simulink model "Step_03"  (Simulink 7.9)
settings: Solver=ode23  StartTime=0.0  StopTime=100  MaxStep=1  RelTol=1e-3
libraries: simulink x1
settings Model: Creator=wcampbel  LastModifiedBy=wcampbel
settings DebuggingCC: FcnCallInpInsideContextMsg=Use local settings  StrictBusMsg=Warning
settings GRTTargetCC: CombineOutputUpdateFcns=off  GRTInterface=on

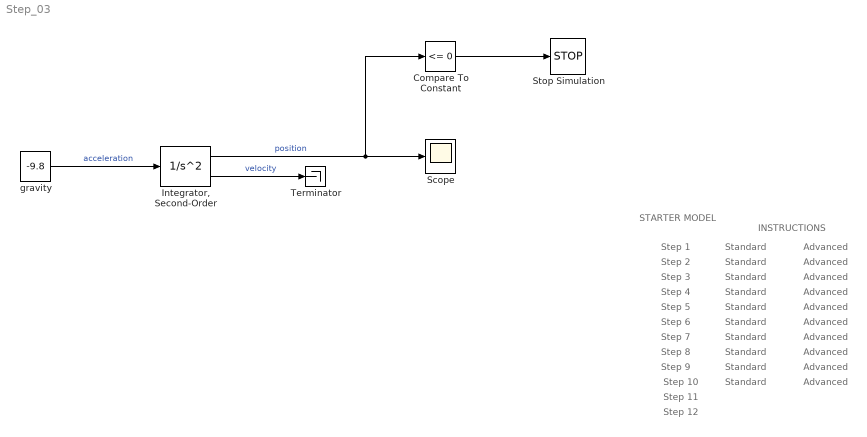
== system Step_03 ==
  note: Step 1
  note: Step 2
  note: Step 3
  note: STARTER
      | MODEL
  note: INSTRUCTIONS
  note: Step 4
  note: Step 5
  note: Step 6
  note: Standard
  note: Advanced
  note: Standard
  note: Advanced
  note: Standard
  note: Advanced
  note: Standard
  note: Standard
  note: Advanced
  note: Standard
  note: Advanced
  note: Step 7
  note: Step 8
  note: Step 9
  note: Step 10
  note: Step 11
  note: Standard
  note: Advanced
  note: Advanced
  note: Advanced
  note: Advanced
  note: Standard
  note: Standard
  note: Standard
  note: Advanced
  note: Step 12
  Compare To Constant : simulink/Logic and Bit Operations/Compare To Constant  relop=<=  const=0  OutDataTypeStr=boolean
  "Integrator, Second-Order" : SecondOrderIntegrator  ICX=500  ICDXDT=5
  Scope : Scope
      settings: TimeRange=12  YMin=-100  YMax=600
  Stop Simulation : Stop
  Terminator : Terminator
  gravity : Constant  Value=-9.8
  wires:
  gravity/1 -> "Integrator, Second-Order"/1  "acceleration"
  "Integrator, Second-Order"/1 -> Scope/1, Compare To Constant/1  "position"
  Compare To Constant/1 -> Stop Simulation/1
  "Integrator, Second-Order"/2 -> Terminator/1  "velocity"
